simulink model "mysql_import_task"  (Simulink 3.00)
libraries: mathlib x1, arclib x1

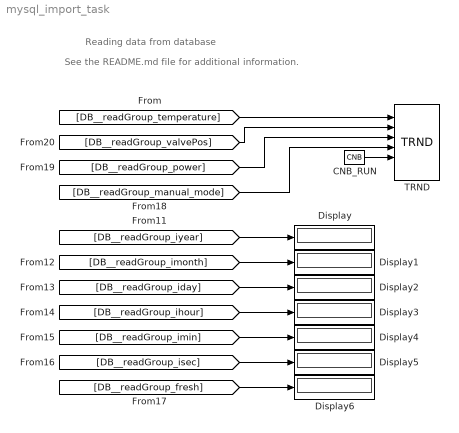
== system mysql_import_task ==
  note: Reading data from database
  note: See the README.md file for additional information.
  CNB_RUN : mathlib/CNB  YCN=on
  Display{,1..6} (7 alike) : Display
      settings: Format=short
  TRND : arclib/TRND  n=4  l=1000  btype=8: Double  ptype1=1: Store  ptype2=1: Store  ptype3=1: Store  ptype4=1: Store  pfac=1  afac=0  arc=0  id=1  Title=Trend Title  timesrc=1
  wires:
  CNB_RUN/1 -> TRND/5
  [DB__readGroup_temperature] -> TRND/1
  [DB__readGroup_iyear] -> Display/1
  [DB__readGroup_imonth] -> Display1/1
  [DB__readGroup_iday] -> Display2/1
  [DB__readGroup_ihour] -> Display3/1
  [DB__readGroup_imin] -> Display4/1
  [DB__readGroup_isec] -> Display5/1
  [DB__readGroup_fresh] -> Display6/1
  [DB__readGroup_manual_mode] -> TRND/4
  [DB__readGroup_power] -> TRND/3
  [DB__readGroup_valvePos] -> TRND/2
